simulink model "angular_velocity"  (R2022b)
settings: Solver=VariableStepAuto  StartTime=0.0  StopTime=500  RelTol=1e-3

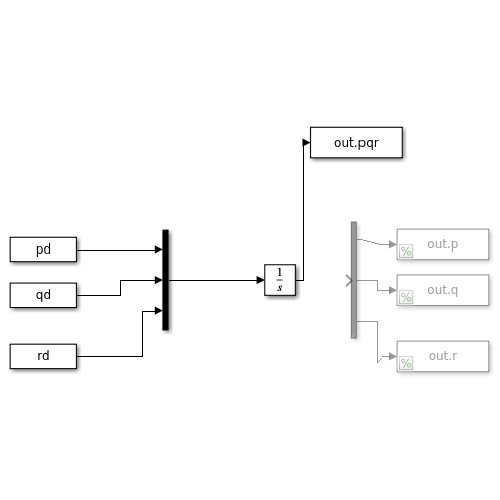
[thumbnail: Simulink's stored preview of the top-level diagram]
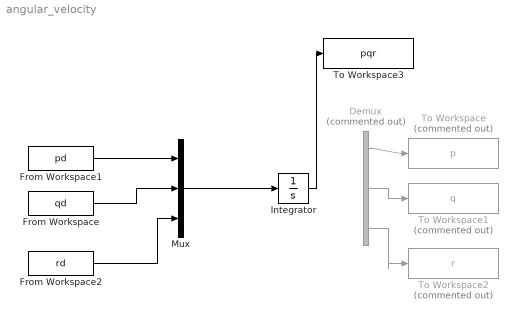
== system angular_velocity ==
  Demux : Demux  Commented=on  Outputs=3
  From Workspace : FromWorkspace  VariableName=qd
  From Workspace1 : FromWorkspace  VariableName=pd
  From Workspace2 : FromWorkspace  VariableName=rd
  Integrator : Integrator
  Mux : Mux  Inputs=3
  To Workspace : ToWorkspace  Commented=on  VariableName=p  SaveFormat=Timeseries  SampleTime=-1
  To Workspace1 : ToWorkspace  Commented=on  VariableName=q  SaveFormat=Timeseries  SampleTime=-1
  To Workspace2 : ToWorkspace  Commented=on  VariableName=r  SaveFormat=Timeseries  SampleTime=-1
  To Workspace3 : ToWorkspace  VariableName=pqr  SaveFormat=Timeseries  SampleTime=-1
  wires:
  Mux/1 -> Integrator/1
  From Workspace1/1 -> Mux/1
  From Workspace/1 -> Mux/2
  From Workspace2/1 -> Mux/3
  Demux/1 -> To Workspace/1
  Demux/2 -> To Workspace1/1
  Demux/3 -> To Workspace2/1
  Integrator/1 -> To Workspace3/1
